simulink library "cassie_lib"  (R2016b)
settings: Solver=VariableStepAuto  StartTime=0.0  StopTime=10.0  RelTol=1e-3
values from neighbouring files (symbols this model uses):
  accel_bias_init = zeros(3,1)    [Copy_of_StateEstimator_RIEKF.m]    (also in Quaternion_EKF.m; RightInvariant_EKF.m; StateEstimator_EKF.m; StateEstimator_RIEKF.m)
  accel_bias_noise_std = 0.1*ones(3,1)    [Copy_of_StateEstimator_RIEKF.m]    (also in Quaternion_EKF.m; RightInvariant_EKF.m; StateEstimator_EKF.m; StateEstimator_RIEKF.m)
  accel_noise_std = 0.1*ones(3,1)    [Copy_of_StateEstimator_RIEKF.m]    (also in Quaternion_EKF.m; RightInvariant_EKF.m; StateEstimator_EKF.m; StateEstimator_RIEKF.m)
  gyro_bias_init = zeros(3,1)    [Copy_of_StateEstimator_RIEKF.m]    (also in Quaternion_EKF.m; RightInvariant_EKF.m; StateEstimator_EKF.m; StateEstimator_RIEKF.m)
  gyro_bias_noise_std = 0.1*ones(3,1)    [Copy_of_StateEstimator_RIEKF.m]    (also in Quaternion_EKF.m; RightInvariant_EKF.m; StateEstimator_EKF.m; StateEstimator_RIEKF.m)
  gyro_noise_std = 0.1*ones(3,1)    [Copy_of_StateEstimator_RIEKF.m]    (also in Quaternion_EKF.m; RightInvariant_EKF.m; StateEstimator_EKF.m; StateEstimator_RIEKF.m)
  X = [R, v, p, dR, dL; 0,0,0,1,0,0,0; 0,0,0,0,1,0,0; 0,0,0,0,0,1,0; 0,0,0,0,0,0,1]    [Copy_of_StateEstimator_RIEKF.m]    (also in RightInvariant_EKF.m; StateEstimator_RIEKF.m)
undefined symbols (not defined in the file or in its folder): A, B, back, cassieParameters, CassieParameters, commands, ControlState, dDown, dLeft, dRight, dUp, EKF_SampleTime, leftBumper, leftStickButton, q_init, rightBumper, rightStickButton, start, v_init, xboxAxes, xboxButtons, xboxPov, Y
libraries: xpcutilitieslib x27, xpcrtudplib x27, dspfdesign x8, simulink x6, slrtlib x3, vrlib x1
(part 2 of 3)

== system cassie_lib/State Estimator Exp Test/Parse Outputs ==
  outputs : Inport
  Bus Selector : BusSelector  OutputSignals=radio
  Parse_Outputs : MATLAB Function  TreatAsAtomicUnit=on
  Send IMU UDP : Subsystem
  Send JointState UDP : Subsystem
  Send Radio : Subsystem
  Send Time : Subsystem
  qwi : Outport
  wi : Outport  Port=2
  ai : Outport  Port=3
  q : Outport  Port=4
  dq : Outport  Port=5
  wires:
  Bus Selector/1 -> Send Radio/1(radio)  "<radio>"
  Parse_Outputs/5(dq) -> dq/1, Send JointState UDP/2(dq)
  outputs/1 -> Bus Selector/1, Parse_Outputs/1(outputs)
  Parse_Outputs/2(wi) -> Send IMU UDP/2(w), wi/1
  Parse_Outputs/4(q) -> q/1, Send JointState UDP/1(q)
  Parse_Outputs/1(qwi) -> qwi/1, Send IMU UDP/1(q)
  Parse_Outputs/3(ai) -> Send IMU UDP/3(a), ai/1

== system cassie_lib/State Estimator Exp Test/Reconstruct State ==
  q_in : Inport
  dq_in : Inport  Port=2
  w : Inport  Port=3
  contact : Inport  Port=4
  mu_in : Inport  Port=5
  ekf_enabled : Inport  Port=6
  Construct_State : MATLAB Function  TreatAsAtomicUnit=on
  Low Pass Filter : Subsystem  TreatAsAtomicUnit=on
  Mux : Mux
  Scope 6 : slrtlib/Displays and Logging/Scope   scopeno=2  scopetype=File  autostart=on  viewmode=Numerical  formatstr='%15.6f'  grid=on  ylimits=[0,0]  nosamples=250  noprepostsamples=0  interleave=1  triggermode=FreeRun  triggersignal=1  trigsignalfromport=on  triggerlevel=0.5  triggerslope=Rising  triggerscope=1  triggersample=0  filename=ekf1.dat  mode=Commit  writesize=512  autorestart=on  dynamicfilemode=off  maxwritefilesize=4000*1024^2
  q : Outport
  dq : Outport  Port=2
  velocity : Outport  Port=3
  wires:
  Low Pass Filter/1(filtered_signal) -> velocity/1
  mu_in/1 -> Construct_State/5(mu), Mux/3
  dq_in/1 -> Construct_State/2("dq ")
  Construct_State/1(q) -> q/1
  Construct_State/3(velocity) -> Mux/1, Low Pass Filter/1(signal)
  Construct_State/5(filter_selector) -> Low Pass Filter/2(selector)
  Mux/1 -> Scope 6/1
  q_in/1 -> Construct_State/1("q ")
  ekf_enabled/1 -> Construct_State/6(ekf_enabled), Mux/4
  Construct_State/2(dq) -> dq/1
  w/1 -> Construct_State/3(w)
  contact/1 -> Construct_State/4(contact)
  Construct_State/4(velocity_kinematic) -> Mux/2

== system cassie_lib/State Estimator Sim Test/Contact Estimator ==
  q : Inport
  GRF_Estimator : MATLAB Function  TreatAsAtomicUnit=on
  Selector : Selector  InputPortWidth=4  IndexOptions=Index vector (dialog)  Indices=[2, 4]  OutputSizes=1
  Send Contact : Subsystem
  GRF : Outport
  contact : Outport  Port=2
  wires:
  GRF_Estimator/1(GRF) -> Selector/1, GRF/1
  GRF_Estimator/2(contact) -> contact/1
  q/1 -> GRF_Estimator/1(q)
  Selector/1 -> Send Contact/1(contact)

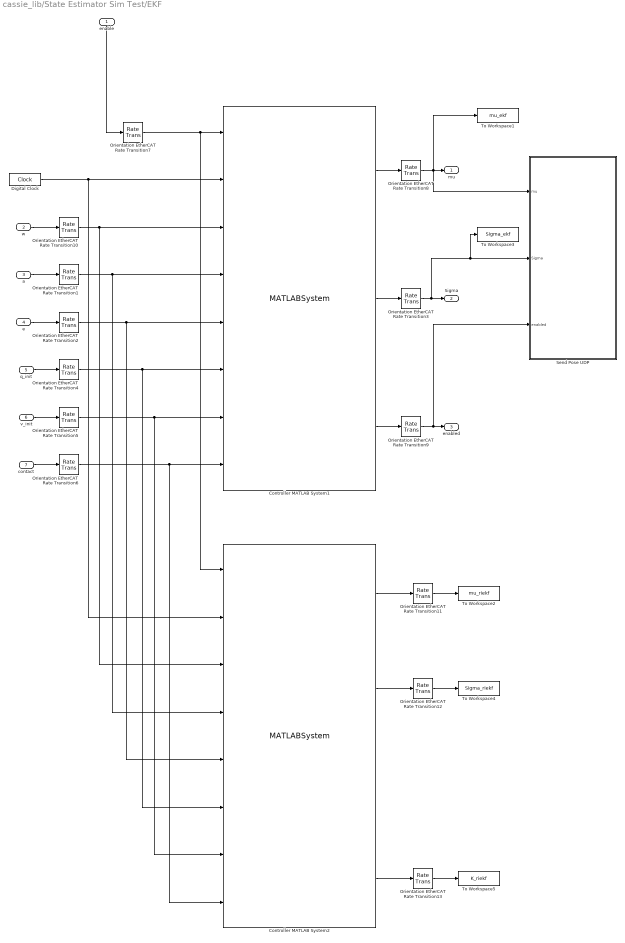
== system cassie_lib/State Estimator Sim Test/EKF ==
  enable : Inport
  w : Inport  Port=2
  a : Inport  Port=3
  e : Inport  Port=4
  q_init : Inport  Port=5
  v_init : Inport  Port=6
  contact : Inport  Port=7
  Controller MATLAB System1 : MATLABSystem  System=StateEstimator_EKF  static_bias_initialization=true  ekf_update_enabled=true  dt=EKF_SampleTime  enable_bias_estimation=enable_bias_estimation  gyro_noise_std=gyro_noise_std  gyro_bias_noise_std=gyro_bias_noise_std  accel_noise_std=accel_noise_std  accel_bias_noise_std=accel_bias_noise_std  contact_noise_std=contact_noise_std  encoder_noise_std=encoder_noise_std  gyro_bias_init=[0;0;0]  accel_bias_init=[0;0;0]  SimulateUsing=Interpreted execution
      mask Type: StateEstimator_EKF
      mask Display:
      | disp('StateEstimator_EKF');
      | port_label('input',1,'EnableFilter');
      | port_label('input',2,'t');
      | port_label('input',3,'w');
      | port_label('input',4,'a');
      | port_label('input',5,'e');
      | port_label('input',6,'q_init');
      | port_label('input',7,'v_init');
      | port_label('input',8,'contact');
      | port_label('output',1,'mu');
      | port_label('output',2,'Sigma');
      | port_label('output',3,'enabled');
  Controller MATLAB System2 : MATLABSystem  System=StateEstimator_RIEKF  static_bias_initialization=true  ekf_update_enabled=true  dt=EKF_SampleTime  enable_bias_estimation=enable_bias_estimation  gyro_noise_std=gyro_noise_std  gyro_bias_noise_std=gyro_bias_noise_std  accel_noise_std=accel_noise_std  accel_bias_noise_std=accel_bias_noise_std  contact_noise_std=contact_noise_std  encoder_noise_std=encoder_noise_std  gyro_bias_init=[0;0;0]  accel_bias_init=[0;0;0]  SimulateUsing=Code generation
      mask Type: StateEstimator_RIEKF
      mask Display:
      | disp('StateEstimator_RIEKF');
      | port_label('input',1,'EnableFilter');
      | port_label('input',2,'t');
      | port_label('input',3,'w');
      | port_label('input',4,'a');
      | port_label('input',5,'e');
      | port_label('input',6,'q_init');
      | port_label('input',7,'v_init');
      | port_label('input',8,'contact');
      | port_label('output',1,'mu');
      | port_label('output',2,'Sigma');
      | port_label('output',3,'enabled');
      | port_label('output',4,'K');
  Digital Clock : DigitalClock  SampleTime=EKF_SampleTime
  Orientation EtherCAT Rate Transition{1..2,4..7,10} (7 alike) : RateTransition  Deterministic=off  OutPortSampleTime=EKF_SampleTime
  Orientation EtherCAT Rate Transition{3,8..9,11..13} (6 alike) : RateTransition  Deterministic=off  OutPortSampleTime=CassieParameters.etherCatSampleTime
  Send Pose UDP : Subsystem
  To Workspace1 : ToWorkspace  VariableName=mu_ekf  SaveFormat=Timeseries  SampleTime=-1
  To Workspace2 : ToWorkspace  VariableName=mu_riekf  SaveFormat=Timeseries  SampleTime=-1
  To Workspace3 : ToWorkspace  VariableName=Sigma_ekf  SaveFormat=Timeseries  SampleTime=-1
  To Workspace4 : ToWorkspace  VariableName=Sigma_riekf  SaveFormat=Timeseries  SampleTime=-1
  To Workspace5 : ToWorkspace  VariableName=K_riekf  SaveFormat=Timeseries  SampleTime=-1
  mu : Outport
  Sigma : Outport  Port=2
  enabled : Outport  Port=3
  wires:
  enable/1 -> Orientation EtherCAT Rate Transition7/1
  Orientation EtherCAT Rate Transition7/1 -> Controller MATLAB System2/1, Controller MATLAB System1/1
  Orientation EtherCAT Rate Transition8/1 -> To Workspace1/1, Send Pose UDP/1(mu), mu/1
  Digital Clock/1 -> Controller MATLAB System2/2, Controller MATLAB System1/2
  Orientation EtherCAT Rate Transition9/1 -> Send Pose UDP/3(enabled), enabled/1
  Controller MATLAB System1/1 -> Orientation EtherCAT Rate Transition8/1
  Controller MATLAB System1/3 -> Orientation EtherCAT Rate Transition9/1
  Orientation EtherCAT Rate Transition6/1 -> Controller MATLAB System2/8, Controller MATLAB System1/8
  Orientation EtherCAT Rate Transition5/1 -> Controller MATLAB System2/7, Controller MATLAB System1/7
  q_init/1 -> Orientation EtherCAT Rate Transition4/1
  v_init/1 -> Orientation EtherCAT Rate Transition5/1
  contact/1 -> Orientation EtherCAT Rate Transition6/1
  w/1 -> Orientation EtherCAT Rate Transition10/1
  Orientation EtherCAT Rate Transition10/1 -> Controller MATLAB System2/3, Controller MATLAB System1/3
  a/1 -> Orientation EtherCAT Rate Transition1/1
  e/1 -> Orientation EtherCAT Rate Transition2/1
  Controller MATLAB System1/2 -> Orientation EtherCAT Rate Transition3/1
  Orientation EtherCAT Rate Transition3/1 -> To Workspace3/1, Send Pose UDP/2(Sigma), Sigma/1
  Orientation EtherCAT Rate Transition1/1 -> Controller MATLAB System2/4, Controller MATLAB System1/4
  Orientation EtherCAT Rate Transition2/1 -> Controller MATLAB System2/5, Controller MATLAB System1/5
  Orientation EtherCAT Rate Transition4/1 -> Controller MATLAB System2/6, Controller MATLAB System1/6
  Controller MATLAB System2/1 -> Orientation EtherCAT Rate Transition11/1
  Orientation EtherCAT Rate Transition11/1 -> To Workspace2/1
  Controller MATLAB System2/2 -> Orientation EtherCAT Rate Transition12/1
  Orientation EtherCAT Rate Transition12/1 -> To Workspace4/1
  Controller MATLAB System2/4 -> Orientation EtherCAT Rate Transition13/1
  Orientation EtherCAT Rate Transition13/1 -> To Workspace5/1

== system cassie_lib/State Estimator Sim Test/Kinematic Velocity Estimator ==
  w : Inport
  q : Inport  Port=2
  dq : Inport  Port=3
  contact : Inport  Port=4
  Kinematic_Velocity : MATLAB Function  TreatAsAtomicUnit=on
  Selector2 : Selector  InputPortWidth=20  IndexOptions=Index vector (dialog)  Indices=[7:20]  OutputSizes=1
  Selector3 : Selector  InputPortWidth=20  IndexOptions=Index vector (dialog)  Indices=[7:20]  OutputSizes=1
  velocity_kinematic : Outport
  wires:
  w/1 -> Kinematic_Velocity/1(w)
  contact/1 -> Kinematic_Velocity/4(contact)
  dq/1 -> Selector3/1
  Kinematic_Velocity/1(velocity) -> velocity_kinematic/1
  q/1 -> Selector2/1
  Selector3/1 -> Kinematic_Velocity/3(e_dot)
  Selector2/1 -> Kinematic_Velocity/2(e)

== system cassie_lib/State Estimator Sim Test/Local Map UDP ==
  note: Local Map UDP Data Structure
      |
      | Map Information
      | double time
      | double resolution
      | double length_x
      | double length_y
      |
      | Map Center Pose
      | double position_x
      | double position_y
      | double position_z
      | double orientation_x
      | double orientation_y
      | double orientation_z
      | double orientation_w
      |
      | Update Block Data
      | double row_start_index
      | double column_start_index
      | double[100] elevation_data
  "Byte Unpacking " : xpcutilitieslib/Byte Unpacking   MaskUnpackedDataTypes={'double'}  MaskUnpackedDataSizes={[45]}  MaskAlignment=1
  Data Store Memory : DataStoreMemory  DataStoreName=local_map  ReadBeforeWriteMsg=warning  WriteAfterWriteMsg=warning  WriteAfterReadMsg=warning  ShowAdditionalParam=off
  Data Store Write : DataStoreWrite  DataStoreName=local_map
  Receive : xpcrtudplib/UDP Receive  ipAddressVal=Use host-target connection  localPort=25000  rcvWidth=45*8  rcvFmAny=off  fmAddress=10.10.10.5  sampleTime=-1
  Terminator : Terminator
  wires:
  Receive/2 -> Terminator/1
  Receive/1 -> "Byte Unpacking "/1
  "Byte Unpacking "/1 -> Data Store Write/1

== system cassie_lib/State Estimator Sim Test/Parse Outputs ==
  outputs : Inport
  Bus Selector : BusSelector  OutputSignals=radio
  Parse_Outputs : MATLAB Function  TreatAsAtomicUnit=on
  Send IMU UDP : Subsystem
  Send JointState UDP : Subsystem
  Send Radio : Subsystem
  Send Time : Subsystem
  qwi : Outport
  wi : Outport  Port=2
  ai : Outport  Port=3
  q : Outport  Port=4
  dq : Outport  Port=5
  wires:
  Bus Selector/1 -> Send Radio/1(radio)  "<radio>"
  Parse_Outputs/5(dq) -> dq/1, Send JointState UDP/2(dq)
  outputs/1 -> Bus Selector/1, Parse_Outputs/1(outputs)
  Parse_Outputs/2(wi) -> Send IMU UDP/2(w), wi/1
  Parse_Outputs/4(q) -> q/1, Send JointState UDP/1(q)
  Parse_Outputs/1(qwi) -> qwi/1, Send IMU UDP/1(q)
  Parse_Outputs/3(ai) -> Send IMU UDP/3(a), ai/1

== system cassie_lib/State Estimator Sim Test/Reconstruct State ==
  q_in : Inport
  dq_in : Inport  Port=2
  w : Inport  Port=3
  contact : Inport  Port=4
  mu_in : Inport  Port=5
  ekf_enabled : Inport  Port=6
  Construct_State : MATLAB Function  TreatAsAtomicUnit=on
  Low Pass Filter : Subsystem  TreatAsAtomicUnit=on
  Mux : Mux
  Scope 6 : slrtlib/Displays and Logging/Scope   scopeno=1  scopetype=File  autostart=on  viewmode=Numerical  formatstr='%15.6f'  grid=on  ylimits=[0,0]  nosamples=250  noprepostsamples=0  interleave=1  triggermode=FreeRun  triggersignal=1  trigsignalfromport=on  triggerlevel=0.5  triggerslope=Rising  triggerscope=1  triggersample=0  filename=ekf.dat  mode=Commit  writesize=512  autorestart=on  dynamicfilemode=off  maxwritefilesize=4000*1024^2
  q : Outport
  dq : Outport  Port=2
  velocity : Outport  Port=3
  wires:
  Low Pass Filter/1(filtered_signal) -> velocity/1
  mu_in/1 -> Construct_State/5(mu), Mux/3
  dq_in/1 -> Construct_State/2("dq ")
  Construct_State/1(q) -> q/1
  Construct_State/3(velocity) -> Mux/1, Low Pass Filter/1(signal)
  Construct_State/5(filter_selector) -> Low Pass Filter/2(selector)
  Mux/1 -> Scope 6/1
  q_in/1 -> Construct_State/1("q ")
  ekf_enabled/1 -> Construct_State/6(ekf_enabled), Mux/4
  Construct_State/2(dq) -> dq/1
  w/1 -> Construct_State/3(w)
  contact/1 -> Construct_State/4(contact)
  Construct_State/4(velocity_kinematic) -> Mux/2

== system cassie_lib/Send UDP Only/Contact Estimator/Send Contact ==
  contact : Inport
  "Byte Packing " : xpcutilitieslib/Byte Packing   MaskPackedDataType=uint8  MaskUnpackedDataTypes={'double'}  MaskAlignment=1
  Digital Clock : DigitalClock  SampleTime=CassieParameters.etherCatSampleTime
  Mux1 : Mux  Inputs=2
  Orientation EtherCAT Rate Transition10 : RateTransition  Deterministic=off  OutPortSampleTime=Contact_UDP_SampleTime
  Send : xpcrtudplib/UDP Send  ipAddressVal=Use host-target connection  localPort=-1  toAddress=10.10.10.5  toPort=25004  sampleTime=Contact_UDP_SampleTime
  Width : Width
  wires:
  Mux1/1 -> Orientation EtherCAT Rate Transition10/1
  "Byte Packing "/1 -> Width/1, Send/1
  Width/1 -> Send/2
  Orientation EtherCAT Rate Transition10/1 -> "Byte Packing "/1
  Digital Clock/1 -> Mux1/1
  contact/1 -> Mux1/2

== system cassie_lib/Send UDP Only/Parse Outputs/Send IMU UDP ==
  q : Inport
  w : Inport  Port=2
  a : Inport  Port=3
  "Byte Packing " : xpcutilitieslib/Byte Packing   MaskPackedDataType=uint8  MaskUnpackedDataTypes={'double'}  MaskAlignment=1
  Digital Clock : DigitalClock  SampleTime=CassieParameters.etherCatSampleTime
  Invert Quaterion for ROS : MATLAB Function  TreatAsAtomicUnit=on
  Mux1 : Mux
  Orientation EtherCAT Rate Transition10 : RateTransition  Deterministic=off  OutPortSampleTime=IMU_UDP_SampleTime
  Send : xpcrtudplib/UDP Send  ipAddressVal=Use host-target connection  localPort=-1  toAddress=10.10.10.5  toPort=25001  sampleTime=IMU_UDP_SampleTime
  Width : Width
  wires:
  Mux1/1 -> Orientation EtherCAT Rate Transition10/1
  "Byte Packing "/1 -> Width/1, Send/1
  Width/1 -> Send/2
  Orientation EtherCAT Rate Transition10/1 -> "Byte Packing "/1
  Digital Clock/1 -> Mux1/1
  a/1 -> Mux1/4
  q/1 -> Invert Quaterion for ROS/1(q)
  w/1 -> Mux1/3
  Invert Quaterion for ROS/1(q_inv) -> Mux1/2

== system cassie_lib/Send UDP Only/Parse Outputs/Send JointState UDP ==
  q : Inport
  dq : Inport  Port=2
  "Byte Packing " : xpcutilitieslib/Byte Packing   MaskPackedDataType=uint8  MaskUnpackedDataTypes={'double'}  MaskAlignment=1
  Digital Clock : DigitalClock  SampleTime=CassieParameters.etherCatSampleTime
  Mux1 : Mux  Inputs=3
  Orientation EtherCAT Rate Transition10 : RateTransition  Deterministic=off  OutPortSampleTime=JointState_UDP_SampleTime
  Parse_Outputs : MATLAB Function  TreatAsAtomicUnit=on
  Send : xpcrtudplib/UDP Send  ipAddressVal=Use host-target connection  localPort=-1  toAddress=10.10.10.5  toPort=25002  sampleTime=JointState_UDP_SampleTime
  Width : Width
  wires:
  Mux1/1 -> Orientation EtherCAT Rate Transition10/1
  "Byte Packing "/1 -> Width/1, Send/1
  Width/1 -> Send/2
  Orientation EtherCAT Rate Transition10/1 -> "Byte Packing "/1
  Digital Clock/1 -> Mux1/1
  Parse_Outputs/1(q_reduced) -> Mux1/2
  Parse_Outputs/2(dq_reduced) -> Mux1/3
  dq/1 -> Parse_Outputs/2(dq)
  q/1 -> Parse_Outputs/1(q)

== system cassie_lib/Send UDP Only/Parse Outputs/Send Radio ==
  radio : Inport
  "Byte Packing " : xpcutilitieslib/Byte Packing   MaskPackedDataType=uint8  MaskUnpackedDataTypes={'double'}  MaskAlignment=1
  Digital Clock : DigitalClock  SampleTime=CassieParameters.etherCatSampleTime
  Mux1 : Mux  Inputs=2
  Orientation EtherCAT Rate Transition10 : RateTransition  Deterministic=off  OutPortSampleTime=Radio_UDP_SampleTime
  Send : xpcrtudplib/UDP Send  ipAddressVal=Use host-target connection  localPort=-1  toAddress=10.10.10.5  toPort=25003  sampleTime=Radio_UDP_SampleTime
  Width : Width
  wires:
  Mux1/1 -> Orientation EtherCAT Rate Transition10/1
  "Byte Packing "/1 -> Width/1, Send/1
  Width/1 -> Send/2
  Orientation EtherCAT Rate Transition10/1 -> "Byte Packing "/1
  Digital Clock/1 -> Mux1/1
  radio/1 -> Mux1/2

== system cassie_lib/Send UDP Only/Parse Outputs/Send Time ==
  "Byte Packing " : xpcutilitieslib/Byte Packing   MaskPackedDataType=uint8  MaskUnpackedDataTypes={'double'}  MaskAlignment=1
  Digital Clock : DigitalClock  SampleTime=CassieParameters.etherCatSampleTime
  Orientation EtherCAT Rate Transition10 : RateTransition  Deterministic=off  OutPortSampleTime=Time_UDP_SampleTime
  Send : xpcrtudplib/UDP Send  ipAddressVal=Use host-target connection  localPort=-1  toAddress=10.10.10.5  toPort=25005  sampleTime=Time_UDP_SampleTime
  Width : Width
  wires:
  Digital Clock/1 -> Orientation EtherCAT Rate Transition10/1
  "Byte Packing "/1 -> Width/1, Send/1
  Width/1 -> Send/2
  Orientation EtherCAT Rate Transition10/1 -> "Byte Packing "/1

== system cassie_lib/State Estimator/Contact Estimator/Send Contact ==
  contact : Inport
  "Byte Packing " : xpcutilitieslib/Byte Packing   MaskPackedDataType=uint8  MaskUnpackedDataTypes={'double'}  MaskAlignment=1
  Digital Clock : DigitalClock  SampleTime=CassieParameters.etherCatSampleTime
  Mux1 : Mux  Inputs=2
  Orientation EtherCAT Rate Transition10 : RateTransition  Deterministic=off  OutPortSampleTime=Contact_UDP_SampleTime
  Send : xpcrtudplib/UDP Send  ipAddressVal=Use host-target connection  localPort=-1  toAddress=10.10.10.5  toPort=25004  sampleTime=Contact_UDP_SampleTime
  Width : Width
  wires:
  Mux1/1 -> Orientation EtherCAT Rate Transition10/1
  "Byte Packing "/1 -> Width/1, Send/1
  Width/1 -> Send/2
  Orientation EtherCAT Rate Transition10/1 -> "Byte Packing "/1
  Digital Clock/1 -> Mux1/1
  contact/1 -> Mux1/2

== system cassie_lib/State Estimator/EKF/Send Pose UDP ==
  mu : Inport
  Sigma : Inport  Port=2
  enabled : Inport  Port=3
  "Byte Packing " : xpcutilitieslib/Byte Packing   MaskPackedDataType=uint8  MaskUnpackedDataTypes={'double'}  MaskAlignment=1
  ConstructPoseData : MATLAB Function  TreatAsAtomicUnit=on
  Digital Clock : DigitalClock  SampleTime=CassieParameters.etherCatSampleTime
  Mux1 : Mux
  Orientation EtherCAT Rate Transition10 : RateTransition  Deterministic=off  OutPortSampleTime=Pose_UDP_SampleTime
  Send : xpcrtudplib/UDP Send  ipAddressVal=Use host-target connection  localPort=-1  toAddress=10.10.10.5  toPort=25000  sampleTime=Pose_UDP_SampleTime
  Width : Width
  wires:
  Mux1/1 -> Orientation EtherCAT Rate Transition10/1
  "Byte Packing "/1 -> Width/1, Send/1
  Width/1 -> Send/2
  Orientation EtherCAT Rate Transition10/1 -> "Byte Packing "/1
  mu/1 -> Mux1/4, ConstructPoseData/1(mu)
  Sigma/1 -> ConstructPoseData/2(Sigma)
  enabled/1 -> Mux1/2
  Digital Clock/1 -> Mux1/1
  ConstructPoseData/1(pose_data) -> Mux1/3

== system cassie_lib/State Estimator/Parse Outputs/Send IMU UDP ==
  q : Inport
  w : Inport  Port=2
  a : Inport  Port=3
  "Byte Packing " : xpcutilitieslib/Byte Packing   MaskPackedDataType=uint8  MaskUnpackedDataTypes={'double'}  MaskAlignment=1
  Digital Clock : DigitalClock  SampleTime=CassieParameters.etherCatSampleTime
  Invert Quaterion for ROS : MATLAB Function  TreatAsAtomicUnit=on
  Mux1 : Mux
  Orientation EtherCAT Rate Transition10 : RateTransition  Deterministic=off  OutPortSampleTime=IMU_UDP_SampleTime
  Send : xpcrtudplib/UDP Send  ipAddressVal=Use host-target connection  localPort=-1  toAddress=10.10.10.5  toPort=25001  sampleTime=IMU_UDP_SampleTime
  Width : Width
  wires:
  Mux1/1 -> Orientation EtherCAT Rate Transition10/1
  "Byte Packing "/1 -> Width/1, Send/1
  Width/1 -> Send/2
  Orientation EtherCAT Rate Transition10/1 -> "Byte Packing "/1
  Digital Clock/1 -> Mux1/1
  a/1 -> Mux1/4
  q/1 -> Invert Quaterion for ROS/1(q)
  w/1 -> Mux1/3
  Invert Quaterion for ROS/1(q_inv) -> Mux1/2

== system cassie_lib/State Estimator/Parse Outputs/Send JointState UDP ==
  q : Inport
  dq : Inport  Port=2
  "Byte Packing " : xpcutilitieslib/Byte Packing   MaskPackedDataType=uint8  MaskUnpackedDataTypes={'double'}  MaskAlignment=1
  Digital Clock : DigitalClock  SampleTime=CassieParameters.etherCatSampleTime
  Mux1 : Mux  Inputs=3
  Orientation EtherCAT Rate Transition10 : RateTransition  Deterministic=off  OutPortSampleTime=JointState_UDP_SampleTime
  Parse_Outputs : MATLAB Function  TreatAsAtomicUnit=on
  Send : xpcrtudplib/UDP Send  ipAddressVal=Use host-target connection  localPort=-1  toAddress=10.10.10.5  toPort=25002  sampleTime=JointState_UDP_SampleTime
  Width : Width
  wires:
  Mux1/1 -> Orientation EtherCAT Rate Transition10/1
  "Byte Packing "/1 -> Width/1, Send/1
  Width/1 -> Send/2
  Orientation EtherCAT Rate Transition10/1 -> "Byte Packing "/1
  Digital Clock/1 -> Mux1/1
  Parse_Outputs/1(q_reduced) -> Mux1/2
  Parse_Outputs/2(dq_reduced) -> Mux1/3
  dq/1 -> Parse_Outputs/2(dq)
  q/1 -> Parse_Outputs/1(q)

== system cassie_lib/State Estimator/Parse Outputs/Send Radio ==
  radio : Inport
  "Byte Packing " : xpcutilitieslib/Byte Packing   MaskPackedDataType=uint8  MaskUnpackedDataTypes={'double'}  MaskAlignment=1
  Digital Clock : DigitalClock  SampleTime=CassieParameters.etherCatSampleTime
  Mux1 : Mux  Inputs=2
  Orientation EtherCAT Rate Transition10 : RateTransition  Deterministic=off  OutPortSampleTime=Radio_UDP_SampleTime
  Send : xpcrtudplib/UDP Send  ipAddressVal=Use host-target connection  localPort=-1  toAddress=10.10.10.5  toPort=25003  sampleTime=Radio_UDP_SampleTime
  Width : Width
  wires:
  Mux1/1 -> Orientation EtherCAT Rate Transition10/1
  "Byte Packing "/1 -> Width/1, Send/1
  Width/1 -> Send/2
  Orientation EtherCAT Rate Transition10/1 -> "Byte Packing "/1
  Digital Clock/1 -> Mux1/1
  radio/1 -> Mux1/2

== system cassie_lib/State Estimator/Parse Outputs/Send Time ==
  "Byte Packing " : xpcutilitieslib/Byte Packing   MaskPackedDataType=uint8  MaskUnpackedDataTypes={'double'}  MaskAlignment=1
  Digital Clock : DigitalClock  SampleTime=CassieParameters.etherCatSampleTime
  Orientation EtherCAT Rate Transition10 : RateTransition  Deterministic=off  OutPortSampleTime=Time_UDP_SampleTime
  Send : xpcrtudplib/UDP Send  ipAddressVal=Use host-target connection  localPort=-1  toAddress=10.10.10.105  toPort=25005  sampleTime=Time_UDP_SampleTime
  Width : Width
  wires:
  Digital Clock/1 -> Orientation EtherCAT Rate Transition10/1
  "Byte Packing "/1 -> Width/1, Send/1
  Width/1 -> Send/2
  Orientation EtherCAT Rate Transition10/1 -> "Byte Packing "/1

== system cassie_lib/State Estimator/Reconstruct State/Low Pass Filter ==
  signal : Inport  Partition=on  PartitionDimension=1  PartitionWidth=1
  selector : Inport  Port=2
  For Each : ForEach  DisableCoverage=on  IndexMode=One-based
  Lowpass Filter : dspfdesign/Lowpass Filter  FilterType=FIR  DesignForMinimumOrder=on  FilterOrder=50  PassbandFrequency=1  StopbandFrequency=10  PassbandRipple=1  StopbandAttenuation=20  InheritSampleRate=off  SampleRate=2000  SimulateUsing=Code generation  roundingMode=Floor  coeffsDataTypeStr=fixdt(1,16)
  Lowpass Filter1 : dspfdesign/Lowpass Filter  FilterType=FIR  DesignForMinimumOrder=on  FilterOrder=50  PassbandFrequency=1  StopbandFrequency=5  PassbandRipple=1  StopbandAttenuation=30  InheritSampleRate=off  SampleRate=2000  SimulateUsing=Code generation  roundingMode=Floor  coeffsDataTypeStr=fixdt(1,16)
  Switch : Switch  Criteria=u2 > Threshold
  filtered_signal : Outport  ConcatenationDimension=1
  wires:
  signal/1 -> Lowpass Filter1/1, Lowpass Filter/1
  selector/1 -> Switch/2
  Switch/1 -> filtered_signal/1
  Lowpass Filter/1 -> Switch/1
  Lowpass Filter1/1 -> Switch/3

== system cassie_lib/State Estimator Exp Test/Contact Estimator/Send Contact ==
  contact : Inport
  "Byte Packing " : xpcutilitieslib/Byte Packing   MaskPackedDataType=uint8  MaskUnpackedDataTypes={'double'}  MaskAlignment=1
  Digital Clock : DigitalClock  SampleTime=CassieParameters.etherCatSampleTime
  Mux1 : Mux  Inputs=2
  Orientation EtherCAT Rate Transition10 : RateTransition  Deterministic=off  OutPortSampleTime=Contact_UDP_SampleTime
  Send : xpcrtudplib/UDP Send  ipAddressVal=Use host-target connection  localPort=-1  toAddress=10.10.10.5  toPort=25004  sampleTime=Contact_UDP_SampleTime
  Width : Width
  wires:
  Mux1/1 -> Orientation EtherCAT Rate Transition10/1
  "Byte Packing "/1 -> Width/1, Send/1
  Width/1 -> Send/2
  Orientation EtherCAT Rate Transition10/1 -> "Byte Packing "/1
  Digital Clock/1 -> Mux1/1
  contact/1 -> Mux1/2

== system cassie_lib/State Estimator Exp Test/EKF/Send Pose UDP ==
  mu : Inport
  Sigma : Inport  Port=2
  enabled : Inport  Port=3
  "Byte Packing " : xpcutilitieslib/Byte Packing   MaskPackedDataType=uint8  MaskUnpackedDataTypes={'double'}  MaskAlignment=1
  ConstructPoseData : MATLAB Function  TreatAsAtomicUnit=on
  Digital Clock : DigitalClock  SampleTime=CassieParameters.etherCatSampleTime
  Mux1 : Mux
  Orientation EtherCAT Rate Transition10 : RateTransition  Deterministic=off  OutPortSampleTime=Pose_UDP_SampleTime
  Send : xpcrtudplib/UDP Send  ipAddressVal=Use host-target connection  localPort=-1  toAddress=10.10.10.5  toPort=25000  sampleTime=Pose_UDP_SampleTime
  Width : Width
  wires:
  Mux1/1 -> Orientation EtherCAT Rate Transition10/1
  "Byte Packing "/1 -> Width/1, Send/1
  Width/1 -> Send/2
  Orientation EtherCAT Rate Transition10/1 -> "Byte Packing "/1
  mu/1 -> Mux1/4, ConstructPoseData/1(mu)
  Sigma/1 -> ConstructPoseData/2(Sigma)
  enabled/1 -> Mux1/2
  Digital Clock/1 -> Mux1/1
  ConstructPoseData/1(pose_data) -> Mux1/3

== system cassie_lib/State Estimator Exp Test/Parse Outputs/Send IMU UDP ==
  q : Inport
  w : Inport  Port=2
  a : Inport  Port=3
  "Byte Packing " : xpcutilitieslib/Byte Packing   MaskPackedDataType=uint8  MaskUnpackedDataTypes={'double'}  MaskAlignment=1
  Digital Clock : DigitalClock  SampleTime=CassieParameters.etherCatSampleTime
  Invert Quaterion for ROS : MATLAB Function  TreatAsAtomicUnit=on
  Mux1 : Mux
  Orientation EtherCAT Rate Transition10 : RateTransition  Deterministic=off  OutPortSampleTime=IMU_UDP_SampleTime
  Send : xpcrtudplib/UDP Send  ipAddressVal=Use host-target connection  localPort=-1  toAddress=10.10.10.5  toPort=25001  sampleTime=IMU_UDP_SampleTime
  Width : Width
  wires:
  Mux1/1 -> Orientation EtherCAT Rate Transition10/1
  "Byte Packing "/1 -> Width/1, Send/1
  Width/1 -> Send/2
  Orientation EtherCAT Rate Transition10/1 -> "Byte Packing "/1
  Digital Clock/1 -> Mux1/1
  a/1 -> Mux1/4
  q/1 -> Invert Quaterion for ROS/1(q)
  w/1 -> Mux1/3
  Invert Quaterion for ROS/1(q_inv) -> Mux1/2

== system cassie_lib/State Estimator Exp Test/Parse Outputs/Send JointState UDP ==
  q : Inport
  dq : Inport  Port=2
  "Byte Packing " : xpcutilitieslib/Byte Packing   MaskPackedDataType=uint8  MaskUnpackedDataTypes={'double'}  MaskAlignment=1
  Digital Clock : DigitalClock  SampleTime=CassieParameters.etherCatSampleTime
  Mux1 : Mux  Inputs=3
  Orientation EtherCAT Rate Transition10 : RateTransition  Deterministic=off  OutPortSampleTime=JointState_UDP_SampleTime
  Parse_Outputs : MATLAB Function  TreatAsAtomicUnit=on
  Send : xpcrtudplib/UDP Send  ipAddressVal=Use host-target connection  localPort=-1  toAddress=10.10.10.5  toPort=25002  sampleTime=JointState_UDP_SampleTime
  Width : Width
  wires:
  Mux1/1 -> Orientation EtherCAT Rate Transition10/1
  "Byte Packing "/1 -> Width/1, Send/1
  Width/1 -> Send/2
  Orientation EtherCAT Rate Transition10/1 -> "Byte Packing "/1
  Digital Clock/1 -> Mux1/1
  Parse_Outputs/1(q_reduced) -> Mux1/2
  Parse_Outputs/2(dq_reduced) -> Mux1/3
  dq/1 -> Parse_Outputs/2(dq)
  q/1 -> Parse_Outputs/1(q)

== system cassie_lib/State Estimator Exp Test/Parse Outputs/Send Radio ==
  radio : Inport
  "Byte Packing " : xpcutilitieslib/Byte Packing   MaskPackedDataType=uint8  MaskUnpackedDataTypes={'double'}  MaskAlignment=1
  Digital Clock : DigitalClock  SampleTime=CassieParameters.etherCatSampleTime
  Mux1 : Mux  Inputs=2
  Orientation EtherCAT Rate Transition10 : RateTransition  Deterministic=off  OutPortSampleTime=Radio_UDP_SampleTime
  Send : xpcrtudplib/UDP Send  ipAddressVal=Use host-target connection  localPort=-1  toAddress=10.10.10.5  toPort=25003  sampleTime=Radio_UDP_SampleTime
  Width : Width
  wires:
  Mux1/1 -> Orientation EtherCAT Rate Transition10/1
  "Byte Packing "/1 -> Width/1, Send/1
  Width/1 -> Send/2
  Orientation EtherCAT Rate Transition10/1 -> "Byte Packing "/1
  Digital Clock/1 -> Mux1/1
  radio/1 -> Mux1/2

== system cassie_lib/State Estimator Exp Test/Parse Outputs/Send Time ==
  "Byte Packing " : xpcutilitieslib/Byte Packing   MaskPackedDataType=uint8  MaskUnpackedDataTypes={'double'}  MaskAlignment=1
  Digital Clock : DigitalClock  SampleTime=CassieParameters.etherCatSampleTime
  Orientation EtherCAT Rate Transition10 : RateTransition  Deterministic=off  OutPortSampleTime=Time_UDP_SampleTime
  Send : xpcrtudplib/UDP Send  ipAddressVal=Use host-target connection  localPort=-1  toAddress=10.10.10.105  toPort=25005  sampleTime=Time_UDP_SampleTime
  Width : Width
  wires:
  Digital Clock/1 -> Orientation EtherCAT Rate Transition10/1
  "Byte Packing "/1 -> Width/1, Send/1
  Width/1 -> Send/2
  Orientation EtherCAT Rate Transition10/1 -> "Byte Packing "/1

== system cassie_lib/State Estimator Exp Test/Reconstruct State/Low Pass Filter ==
  signal : Inport  Partition=on  PartitionDimension=1  PartitionWidth=1
  selector : Inport  Port=2
  For Each : ForEach  DisableCoverage=on  IndexMode=One-based
  Lowpass Filter : dspfdesign/Lowpass Filter  FilterType=FIR  DesignForMinimumOrder=on  FilterOrder=50  PassbandFrequency=1  StopbandFrequency=10  PassbandRipple=1  StopbandAttenuation=20  InheritSampleRate=off  SampleRate=2000  SimulateUsing=Code generation  roundingMode=Floor  coeffsDataTypeStr=fixdt(1,16)
  Lowpass Filter1 : dspfdesign/Lowpass Filter  FilterType=FIR  DesignForMinimumOrder=on  FilterOrder=50  PassbandFrequency=1  StopbandFrequency=5  PassbandRipple=1  StopbandAttenuation=30  InheritSampleRate=off  SampleRate=2000  SimulateUsing=Code generation  roundingMode=Floor  coeffsDataTypeStr=fixdt(1,16)
  Switch : Switch  Criteria=u2 > Threshold
  filtered_signal : Outport  ConcatenationDimension=1
  wires:
  signal/1 -> Lowpass Filter1/1, Lowpass Filter/1
  selector/1 -> Switch/2
  Switch/1 -> filtered_signal/1
  Lowpass Filter/1 -> Switch/1
  Lowpass Filter1/1 -> Switch/3

== system cassie_lib/State Estimator Sim Test/Contact Estimator/Send Contact ==
  contact : Inport
  "Byte Packing " : xpcutilitieslib/Byte Packing   MaskPackedDataType=uint8  MaskUnpackedDataTypes={'double'}  MaskAlignment=1
  Digital Clock : DigitalClock  SampleTime=CassieParameters.etherCatSampleTime
  Mux1 : Mux  Inputs=2
  Orientation EtherCAT Rate Transition10 : RateTransition  Deterministic=off  OutPortSampleTime=Contact_UDP_SampleTime
  Send : xpcrtudplib/UDP Send  ipAddressVal=Use host-target connection  localPort=-1  toAddress=10.10.10.5  toPort=25004  sampleTime=Contact_UDP_SampleTime
  Width : Width
  wires:
  Mux1/1 -> Orientation EtherCAT Rate Transition10/1
  "Byte Packing "/1 -> Width/1, Send/1
  Width/1 -> Send/2
  Orientation EtherCAT Rate Transition10/1 -> "Byte Packing "/1
  Digital Clock/1 -> Mux1/1
  contact/1 -> Mux1/2

== system cassie_lib/State Estimator Sim Test/EKF/Send Pose UDP ==
  mu : Inport
  Sigma : Inport  Port=2
  enabled : Inport  Port=3
  "Byte Packing " : xpcutilitieslib/Byte Packing   MaskPackedDataType=uint8  MaskUnpackedDataTypes={'double'}  MaskAlignment=1
  ConstructPoseData : MATLAB Function  TreatAsAtomicUnit=on
  Digital Clock : DigitalClock  SampleTime=CassieParameters.etherCatSampleTime
  Mux1 : Mux
  Orientation EtherCAT Rate Transition10 : RateTransition  Deterministic=off  OutPortSampleTime=Pose_UDP_SampleTime
  Send : xpcrtudplib/UDP Send  ipAddressVal=Use host-target connection  localPort=-1  toAddress=10.10.10.5  toPort=25000  sampleTime=Pose_UDP_SampleTime
  Width : Width
  wires:
  Mux1/1 -> Orientation EtherCAT Rate Transition10/1
  "Byte Packing "/1 -> Width/1, Send/1
  Width/1 -> Send/2
  Orientation EtherCAT Rate Transition10/1 -> "Byte Packing "/1
  mu/1 -> Mux1/4, ConstructPoseData/1(mu)
  Sigma/1 -> ConstructPoseData/2(Sigma)
  enabled/1 -> Mux1/2
  Digital Clock/1 -> Mux1/1
  ConstructPoseData/1(pose_data) -> Mux1/3

== system cassie_lib/State Estimator Sim Test/Parse Outputs/Send IMU UDP ==
  q : Inport
  w : Inport  Port=2
  a : Inport  Port=3
  "Byte Packing " : xpcutilitieslib/Byte Packing   MaskPackedDataType=uint8  MaskUnpackedDataTypes={'double'}  MaskAlignment=1
  Digital Clock : DigitalClock  SampleTime=CassieParameters.etherCatSampleTime
  Invert Quaterion for ROS : MATLAB Function  TreatAsAtomicUnit=on
  Mux1 : Mux
  Orientation EtherCAT Rate Transition10 : RateTransition  Deterministic=off  OutPortSampleTime=IMU_UDP_SampleTime
  Send : xpcrtudplib/UDP Send  ipAddressVal=Use host-target connection  localPort=-1  toAddress=10.10.10.5  toPort=25001  sampleTime=IMU_UDP_SampleTime
  Width : Width
  wires:
  Mux1/1 -> Orientation EtherCAT Rate Transition10/1
  "Byte Packing "/1 -> Width/1, Send/1
  Width/1 -> Send/2
  Orientation EtherCAT Rate Transition10/1 -> "Byte Packing "/1
  Digital Clock/1 -> Mux1/1
  a/1 -> Mux1/4
  q/1 -> Invert Quaterion for ROS/1(q)
  w/1 -> Mux1/3
  Invert Quaterion for ROS/1(q_inv) -> Mux1/2

== system cassie_lib/State Estimator Sim Test/Parse Outputs/Send JointState UDP ==
  q : Inport
  dq : Inport  Port=2
  "Byte Packing " : xpcutilitieslib/Byte Packing   MaskPackedDataType=uint8  MaskUnpackedDataTypes={'double'}  MaskAlignment=1
  Digital Clock : DigitalClock  SampleTime=CassieParameters.etherCatSampleTime
  Mux1 : Mux  Inputs=3
  Orientation EtherCAT Rate Transition10 : RateTransition  Deterministic=off  OutPortSampleTime=JointState_UDP_SampleTime
  Parse_Outputs : MATLAB Function  TreatAsAtomicUnit=on
  Send : xpcrtudplib/UDP Send  ipAddressVal=Use host-target connection  localPort=-1  toAddress=10.10.10.5  toPort=25002  sampleTime=JointState_UDP_SampleTime
  Width : Width
  wires:
  Mux1/1 -> Orientation EtherCAT Rate Transition10/1
  "Byte Packing "/1 -> Width/1, Send/1
  Width/1 -> Send/2
  Orientation EtherCAT Rate Transition10/1 -> "Byte Packing "/1
  Digital Clock/1 -> Mux1/1
  Parse_Outputs/1(q_reduced) -> Mux1/2
  Parse_Outputs/2(dq_reduced) -> Mux1/3
  dq/1 -> Parse_Outputs/2(dq)
  q/1 -> Parse_Outputs/1(q)

== system cassie_lib/State Estimator Sim Test/Parse Outputs/Send Radio ==
  radio : Inport
  "Byte Packing " : xpcutilitieslib/Byte Packing   MaskPackedDataType=uint8  MaskUnpackedDataTypes={'double'}  MaskAlignment=1
  Digital Clock : DigitalClock  SampleTime=CassieParameters.etherCatSampleTime
  Mux1 : Mux  Inputs=2
  Orientation EtherCAT Rate Transition10 : RateTransition  Deterministic=off  OutPortSampleTime=Radio_UDP_SampleTime
  Send : xpcrtudplib/UDP Send  ipAddressVal=Use host-target connection  localPort=-1  toAddress=10.10.10.5  toPort=25003  sampleTime=Radio_UDP_SampleTime
  Width : Width
  wires:
  Mux1/1 -> Orientation EtherCAT Rate Transition10/1
  "Byte Packing "/1 -> Width/1, Send/1
  Width/1 -> Send/2
  Orientation EtherCAT Rate Transition10/1 -> "Byte Packing "/1
  Digital Clock/1 -> Mux1/1
  radio/1 -> Mux1/2

== system cassie_lib/State Estimator Sim Test/Parse Outputs/Send Time ==
  "Byte Packing " : xpcutilitieslib/Byte Packing   MaskPackedDataType=uint8  MaskUnpackedDataTypes={'double'}  MaskAlignment=1
  Digital Clock : DigitalClock  SampleTime=CassieParameters.etherCatSampleTime
  Orientation EtherCAT Rate Transition10 : RateTransition  Deterministic=off  OutPortSampleTime=Time_UDP_SampleTime
  Send : xpcrtudplib/UDP Send  ipAddressVal=Use host-target connection  localPort=-1  toAddress=10.10.10.105  toPort=25005  sampleTime=Time_UDP_SampleTime
  Width : Width
  wires:
  Digital Clock/1 -> Orientation EtherCAT Rate Transition10/1
  "Byte Packing "/1 -> Width/1, Send/1
  Width/1 -> Send/2
  Orientation EtherCAT Rate Transition10/1 -> "Byte Packing "/1

== system cassie_lib/State Estimator Sim Test/Reconstruct State/Low Pass Filter ==
  signal : Inport  Partition=on  PartitionDimension=1  PartitionWidth=1
  selector : Inport  Port=2
  For Each : ForEach  DisableCoverage=on  IndexMode=One-based
  Lowpass Filter : dspfdesign/Lowpass Filter  FilterType=FIR  DesignForMinimumOrder=on  FilterOrder=50  PassbandFrequency=1  StopbandFrequency=10  PassbandRipple=1  StopbandAttenuation=20  InheritSampleRate=off  SampleRate=2000  SimulateUsing=Code generation  roundingMode=Floor  coeffsDataTypeStr=fixdt(1,16)
  Lowpass Filter1 : dspfdesign/Lowpass Filter  FilterType=FIR  DesignForMinimumOrder=on  FilterOrder=50  PassbandFrequency=1  StopbandFrequency=5  PassbandRipple=1  StopbandAttenuation=30  InheritSampleRate=off  SampleRate=2000  SimulateUsing=Code generation  roundingMode=Floor  coeffsDataTypeStr=fixdt(1,16)
  Switch : Switch  Criteria=u2 > Threshold
  filtered_signal : Outport  ConcatenationDimension=1
  wires:
  signal/1 -> Lowpass Filter1/1, Lowpass Filter/1
  selector/1 -> Switch/2
  Switch/1 -> filtered_signal/1
  Lowpass Filter/1 -> Switch/1
  Lowpass Filter1/1 -> Switch/3

== matlab function cassie_lib/State Estimator/Parse Outputs/Parse_Outputs ==
  data: qwi output; wi output; ai output; q output; outputs input; dq output
function [qwi, wi, ai, q, dq] = Parse_Outputs(outputs)
%
% Frames:
%   W - Cassie World (inertial frame North-West-Up)
%   N - IMU World (inertial frame North-East-Down)
%   B - Body (cassie pelvis)
%   I - IMU (cassie vectorNav)
%   
%   Author: Ross Hartley 
%   Date:   11/06/2017
%

% Parse IMU Data from the VectorNav on Cassie
cassieOutputs = CassieOutputs;
cassieOutputs.setStructure(outputs);

% IMU Data
% VectorNav outputs quaternion as qin = [qw; qx; qy; qz]
qin = cassieOutputs.getVectorNavOrientation; qin = qin([2,3,4,1]); % Convert to [qx; qy; qz; qw] format
wi = cassieOutputs.getVectorNavAngularVelocity;      % {I}_\omega_{NI}   or   {I}_\omega_{WI}
ai = cassieOutputs.getVectorNavLinearAcceleration;   % {I}_a_{NI}        or   {I}_a_{WI}
Rni = Angles.Quaternion_to_Rotation(qin)'; % R_{NI}
Rbi = R_VectorNav_to_Pelvis(zeros(14,1))';    % R_{BI} 
Rwn = Angles.Rx(pi);                % R_{WN}
Rwi = Rwn*Rni;                      % R_{WI}
Rwb = Rwi*Rbi';                     % R_{WB}
qwi = Angles.Rotation_to_Quaternion(Rwi);
 
% Compute angular velocity of body frame:
%      {I}_\omega_{NI} = {I}_\omega_{NW} + {I}_\omega_{WB} + {I}_\omega_{BI}
%                      =        0        + {I}_\omega_{WB} +       0
%  =>  {B}_\omega_{WB} = R_{BI} * {I}_\omega_{NI}
wb = Rbi*wi; % {B}_\omega_{WB}

% Get positions
qq = Angles.Rotation_to_Euler(Rwb);
qaR = cassieOutputs.getRightLegMotorPositions;
qjR =  cassieOutputs.getRightLegJointPositions;
qaL = cassieOutputs.getLeftLegMotorPositions;
qjL =  cassieOutputs.getLeftLegJointPositions;

% Get velocities
dqq = Angles.AngularVelocity_to_EulerRates(qq, wb);
dqaR = cassieOutputs.getRightLegMotorVelocities;
dqjR =  cassieOutputs.getRightLegJointVelocities;
dqaL = cassieOutputs.getLeftLegMotorVelocities;
dqjL =  cassieOutputs.getLeftLegJointVelocities;

% Construct State Vector
q = [zeros(3,1); qq; qaL(1:3); qaL(4); qjL(1); qjL(2); qaL(5); qaR(1:3); qaR(4); qjR(1); qjR(2); qaR(5)];
dq = [zeros(3,1); dqq; dqaL(1:3); dqaL(4); dqjL(1); dqjL(2); dqaL(5); dqaR(1:3); dqaR(4); dqjR(1); dqjR(2); dqaR(5)];

end

== matlab function cassie_lib/State Estimator/Contact Estimator/GRF_Estimator ==
  data: q input; GRF output; contact output
function [GRF, contact] = GRF_Estimator(q)
% Estimates the ground reaction force in the body frame of the robot
%
% Fe_i = (S_i * J_i^T)^{-1} * S_i * \tau_d
%
J_pR = J_RightToeBottom([zeros(6,1); q(7:end)]);
J_pL = J_LeftToeBottom([zeros(6,1); q(7:end)]);

qs_knee_L = q(11);
qs_tarsus_L = q(10) + q(11) + q(12) - deg2rad(13);

qs_knee_R = q(18);
qs_tarsus_R = q(17) + q(18) + q(19) - deg2rad(13);

tau_L = -[1500; 1250].*[qs_knee_L + qs_tarsus_L; qs_tarsus_L];
tau_R = -[1500; 1250].*[qs_knee_R + qs_tarsus_R; qs_tarsus_R];

GRF_L = -[J_pL([1,3],11), J_pL([1,3],12)] \ tau_L;
GRF_R = -[J_pR([1,3],18), J_pR([1,3],19)] \ tau_R;
GRF = [GRF_L; GRF_R];

% Detect contact using GRF
cL = scaleFactor(GRF(2), 50, 100);
cR = scaleFactor(GRF(4), 50, 100);
contact = [cL; cR];

end

== matlab function cassie_lib/Radio Parser/radio_cmd_assigner ==
  data: ControlStateIn input; radio input; ControlStateOut output Bus: cassieControlStateBus
function ControlStateOut = radio_cmd_assigner(ControlStateIn, radio) %#codegen
%% Copyright 2017 - Ross Hartley

ControlStateOut = ControlStateIn;

%% ON / OFF Commands 

% Shutdown / Pause Time
switch radio.SE
    case -1
        ControlStateOut.commands.shutdown = 1;
        ControlStateOut.commands.pauseTime = 1;
    case 0
        ControlStateOut.commands.shutdown = 0;
        ControlStateOut.commands.pauseTime = 1;
    case 1
        ControlStateOut.commands.shutdown = 0;
        ControlStateOut.commands.pauseTime = 0;        
    otherwise
        ControlStateOut.commands.shutdown = 1;
        ControlStateOut.commands.pauseTime = 1;  
end

% Enable EKF
if radio.SF == 1
	ControlStateOut.commands.EnableEKF = 1;
end

% Scale torque
ControlStateOut.scaling.torque = abs(radio.S1);

% Scale Gait Step Time
ControlStateOut.commands.timeScale = abs(radio.S2);
ControlStateOut.commands.phi = radio.RV;


%% Velocity and Turning Commands

% Turning Command
if ControlStateIn.options.enableTurningCommand
    % Parse right joystick for turning rate (deltaYaw per step)
    ControlStateOut.commands.deltaYaw = -deg2rad(10)*radio.RH;
end


if ControlStateIn.options.enableSagittalVelocityCommand
    % Parse left joystick data for Y Velocity
%     dy_cmd = max(min(radio.LV, 0.8), -0.8);
	dy_cmd = radio.LV*0.8;
    if abs(dy_cmd) < 0.1
        dy_cmd = 0; % Ignore small values
    end
else
    dy_cmd = 0;
end
    
if ControlStateIn.options.enableLateralVelocityCommand
    % Parse right joystick data for X Velocity
%     dx_cmd = max(min(radio.LH, 0.2), -0.2);
	dx_cmd = radio.LH*0.2;
    if abs(dx_cmd) < 0.1
        dx_cmd = 0; % Ignore small values
    end
else
    dx_cmd = 0;
end

% Desired velocity Command
ControlStateOut.commands.velocityDesired = [dy_cmd; dx_cmd; 0];

%% Foot Placement Gain Scaling
% ControlStateOut.scaling.kp_sla = 1*abs(radio.LS);
% ControlStateOut.scaling.kp_sha = 1*abs(radio.RS);

%% Offsets
% ControlStateOut.offsets.st_legLength = 0.1*radio.S2;

%% Tests
if radio.SB == 1
    ControlStateOut.tests.useOptimization = 1;
else
    ControlStateOut.tests.useOptimization = 0;
end

end

== matlab function cassie_lib/Radio Parser/radio_parser ==
  data: outputs input; radio output Bus: radioBus
function radio = radio_parser(outputs) %#codegen
%% Copyright 2017 - Ross Hartley

radio.LV = outputs.radio(1);
radio.LH = outputs.radio(2);
radio.RV = outputs.radio(3);
radio.RH = outputs.radio(4);
radio.S1 = outputs.radio(5);
radio.S2 = outputs.radio(6);
radio.LS = outputs.radio(7);
radio.RS = outputs.radio(8);
radio.SA = outputs.radio(9);
radio.SB = outputs.radio(10);
radio.SC = outputs.radio(11);
radio.SD = outputs.radio(12);
radio.SE = outputs.radio(13);
radio.SF = outputs.radio(14);
radio.SG = outputs.radio(15);
radio.SH = outputs.radio(16);


end

== matlab function cassie_lib/State Estimator/Parse Outputs/Send IMU UDP/Invert Quaterion for ROS ==
  data: q input; q_inv output
function q_inv = fcn(q)
    q_inv = Angles.Rotation_to_Quaternion( Angles.Quaternion_to_Rotation(q)' );
end

== matlab function cassie_lib/Radio Spoofer/radio_cmd_assigner ==
  data: ControlStateIn input; radio input; ControlStateOut output Bus: cassieControlStateBus
function ControlStateOut = radio_cmd_assigner(ControlStateIn, radio) %#codegen
%% Copyright 2017 - Ross Hartley

ControlStateOut = ControlStateIn;

%% ON / OFF Commands 

% Shutdown / Pause Time
switch radio.SE
    case -1
        ControlStateOut.commands.shutdown = 1;
        ControlStateOut.commands.pauseTime = 1;
    case 0
        ControlStateOut.commands.shutdown = 0;
        ControlStateOut.commands.pauseTime = 1;
    case 1
        ControlStateOut.commands.shutdown = 0;
        ControlStateOut.commands.pauseTime = 0;        
    otherwise
        ControlStateOut.commands.shutdown = 1;
        ControlStateOut.commands.pauseTime = 1;  
end

% Enable EKF
if radio.SF == 1
	ControlStateOut.commands.EnableEKF = 1;
end

% Scale torque
ControlStateOut.scaling.torque = abs(radio.S1);

% Scale Gait Step Time
ControlStateOut.commands.timeScale = abs(radio.S2);
ControlStateOut.commands.phi = radio.RV;


%% Velocity and Turning Commands

% Turning Command
if ControlStateIn.options.enableTurningCommand
    % Parse right joystick for turning rate (deltaYaw per step)
    ControlStateOut.commands.deltaYaw = -deg2rad(10)*radio.RH;
end


if ControlStateIn.options.enableSagittalVelocityCommand
    % Parse left joystick data for Y Velocity
%     dy_cmd = max(min(radio.LV, 0.8), -0.8);
	dy_cmd = radio.LV*0.8;
    if abs(dy_cmd) < 0.1
        dy_cmd = 0; % Ignore small values
    end
else
    dy_cmd = 0;
end
    
if ControlStateIn.options.enableLateralVelocityCommand
    % Parse right joystick data for X Velocity
%     dx_cmd = max(min(radio.LH, 0.2), -0.2);
	dx_cmd = radio.LH*0.2;
    if abs(dx_cmd) < 0.1
        dx_cmd = 0; % Ignore small values
    end
else
    dx_cmd = 0;
end

% Desired velocity Command
ControlStateOut.commands.velocityDesired = [dy_cmd; dx_cmd; 0];

%% Foot Placement Gain Scaling
% ControlStateOut.scaling.kp_sla = 1*abs(radio.LS);
% ControlStateOut.scaling.kp_sha = 1*abs(radio.RS);

%% Offsets
% ControlStateOut.offsets.st_legLength = 0.1*radio.S2;

%% Tests
if radio.SB == 1
    ControlStateOut.tests.useOptimization = 1;
else
    ControlStateOut.tests.useOptimization = 0;
end

end

== matlab function cassie_lib/State Estimator/Reconstruct State/Construct_State ==
  data: q output; dq output; q input; dq input; w input; contact input; mu input; ekf_enabled input; velocity output; velocity_kinematic output; filter_selector output
function [q, dq, velocity, velocity_kinematic, filter_selector] = Construct_State(q, dq, w, contact, mu, ekf_enabled)
% Construct state vector and body velocity estimate using raw data and ekf
%   
%   Inputs:
%       q           - state position vector
%       dq          - state velocity vector
%       w           - angular velocity, {I}_\omega_{WI}
%       contact     - contact indicator
%       mu          - EKF state estimate
%       ekf_enabled - EKF enable flag
%
%   Outputs:
%       q                   - 
%       dq                  - 
%       velocity            - EKF body velocity, {W}_v_{WB} 
%       velocity_kinematic  - Kinematic body velocity, {B}_v_{WB} 
%       filter_selector     - used to select low pass filter type
%
%
%   Author: Ross Hartley
%   Date:   11/07/2017

%% Settings
use_ekf_position = true;
use_ekf_orientation = false;
use_ekf_velocity = false;

%% Compute kinematic velocity
e = q(7:end);
e_dot = dq(7:end);

if contact(1) == 1
    pL = p_VectorNav_to_LeftToeBottom(e); % {I}_p_{IL}
    J_pL = J_VectorNav_to_LeftToeBottom(e);
    velocity_kinematic = -J_pL(1:3,:)*e_dot - Angles.skew(w)*pL(1:3,:); % {I}_v_{WI}
elseif contact(2) == 1
    pR = p_VectorNav_to_RightToeBottom(e); % {I}_p_{IR}
    J_pR = J_VectorNav_to_RightToeBottom(e);
    velocity_kinematic = -J_pR(1:3,:)*e_dot - Angles.skew(w)*pR(1:3,:); % {I}_v_{WI}
else
    velocity_kinematic = zeros(3,1);
end

%% Reconstruct State
Rbi = R_VectorNav_to_Pelvis(e)';    % R_{BI}

% Position
if use_ekf_position && ekf_enabled
    Rwi = Angles.Quaternion_to_Rotation(mu(7:10))';
    % {W}_p_{WB} =  {W}_p_{WI} +  {W}_p_{IB}
    q(1:3) = mu(1:3) + Rwi * p_VectorNav_to_Pelvis(e); 
end
 
% Orientation
if use_ekf_orientation && ekf_enabled
    Rwi = Angles.Quaternion_to_Rotation(mu(7:10))';
    Rwb = Rwi * Rbi';
    q(4:6) = Angles.Rotation_to_Euler( Rwb );
end

% Velocity
if use_ekf_velocity && ekf_enabled
    Rwi = Angles.Quaternion_to_Rotation(mu(7:10))';
    Rwb = Rwi * Rbi';
    % {W}_v_{WB} =  {W}_v_{WI} + R_{WI} * skew({I}_w_{WI}) * {I}_p_{IB}
    dq(1:3) = mu(4:6) + Rwi * Angles.skew(w) * p_VectorNav_to_Pelvis(e); 
    % {B}_v_{WB} = R_{BW} * {W}_v_{WB}
    velocity = Rwb' * dq(1:3);
    filter_selector = 1;
else
    Rwb = Angles.Euler_to_Rotation(q(4:6));
    Rwi = Rwb * Rbi;
    % {W}_v_{WB} =  R_{WI} * {I}_v_{WI} + R_{WI} * skew({I}_w_{WI}) * {I}_p_{IB}
    dq(1:3) = Rwi * velocity_kinematic + Rwi * Angles.skew(w) * p_VectorNav_to_Pelvis(e); 
    % {B}_v_{WB} = R_{BW} * {W}_v_{WB}
    velocity = Rwb' * dq(1:3);
    filter_selector = 0;
end



end

== matlab function cassie_lib/State Estimator/Parse Outputs/Send JointState UDP/Parse_Outputs ==
  data: q_reduced output; dq_reduced output; q input; dq input
function [q_reduced, dq_reduced] = ReduceState(q, dq)
% Reduce state vector for use in ROS network

q_reduced = q(7:end);
dq_reduced = dq(7:end);

end

== matlab function cassie_lib/State Estimator/EKF/Send Pose UDP/ConstructPoseData ==
  data: pose_data output; mu input; Sigma input
function pose_data = ConstructPoseData(mu, Sigma)
% Construct pose data for use in ROS network
% Publish everything in pelvis frame
Rwi = Angles.Quaternion_to_Rotation(mu(7:10))';

pose_data = zeros(43,1); 
pose_data(1:3) = mu(1:3) + Rwi*p_VectorNav_to_Pelvis(zeros(14,1));
pose_data(4:7) = Angles.Rotation_to_Quaternion( (Rwi * R_VectorNav_to_Pelvis(zeros(14,1)))' );

% TODO: Convert covariance of IMU pose to Body pose (Ross) 
pose_data(8:end) = reshape(Sigma([1:3,1:3],[7:9,7:9]),[],1);

end
